simulink model "ODIN_Dynamics"  (R2025b)
settings: Solver=VariableStepAuto  StartTime=0.0  StopTime=10.0  RelTol=1e-3
settings Model: Creator=vulcangrip  LastModifiedBy=vulcangrip

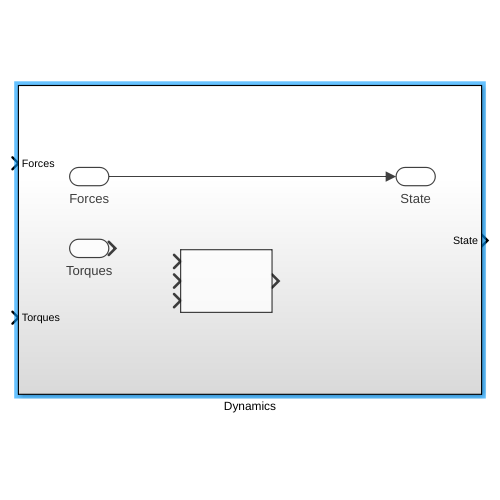
[thumbnail: Simulink's stored preview of the top-level diagram]
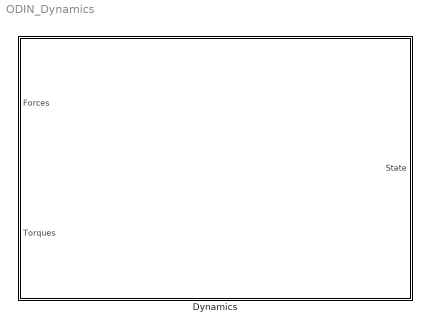
== system ODIN_Dynamics ==
  Dynamics : Subsystem

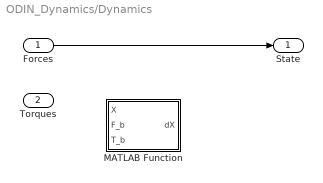
== system ODIN_Dynamics/Dynamics ==
  Forces : Inport
  Torques : Inport  Port=2
  MATLAB Function : MATLAB Function  TreatAsAtomicUnit=on
  State : Outport
  wires:
  Forces/1 -> State/1

== matlab function ODIN_Dynamics/Dynamics/MATLAB Function ==
  data: X input; F_b input; T_b input; dX output
function dX =  fcn(X,F_b,T_b)

dX = odin_dyn(X,F_b,T_b);
